simulink model "tgov1"  (R2014b)
settings: Solver=ode4  StartTime=0.0  StopTime=30  FixedStep=30/100  RelTol=1e-3  EnableMultiTasking=on
values from neighbouring files (symbols this model uses):
  delta_w = 0.0    (= 0)    [tgov1_test.m]
  Dt = 0.0    (= 0)    [tgov1_test.m]
  Pref = .50    (= 0.5)    [tgov1_test.m]
  R = 0.05    [tgov1_test.m]
  T1 = 0.5    [tgov1_test.m]
  T2 = 3.0    (= 3)    [tgov1_test.m]
  T3 = 10.0    (= 10)    [tgov1_test.m]
settings Model: Creator=thad  LastModifiedBy=heyth
settings OptimizationCC: UseDivisionForNetSlopeComputation=off  SimCompilerOptimization=off
settings DebuggingCC: FcnCallInpInsideContextMsg=error  FrameProcessingCompatibilityMsg=error  SFExecutionAtInitializationDiag=none
settings HardwareCC: ProdBitPerSizeT=32  ProdBitPerPtrDiffT=32
settings RTWCC: RTWCompilerOptimization=off
settings ConfigComp: CovMetricSettings=dw  CovHtmlReporting=on  CovSaveCumulativeToWorkspaceVar=on  CovSaveSingleToWorkspaceVar=on  CovExternalEMLEnable=off  CovSFcnEnable=off

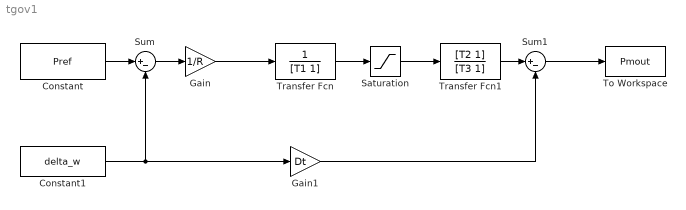
== system tgov1 ==
  Constant : Constant  Value=Pref
  Constant1 : Constant  Value=delta_w
  Gain : Gain  Gain=1/R
  Gain1 : Gain  Gain=Dt
  Saturation : Saturate  UpperLimit=1  LowerLimit=0
  Sum : Sum  Inputs=|+-
  Sum1 : Sum  Inputs=|+-
  To Workspace : ToWorkspace  VariableName=Pmout  SampleTime=-1
  Transfer Fcn : TransferFcn  Denominator=[T1 1]
  Transfer Fcn1 : TransferFcn  Numerator=[T2 1]  Denominator=[T3 1]
  wires:
  Constant1/1 -> Sum/2, Gain1/1
  Transfer Fcn/1 -> Saturation/1
  Saturation/1 -> Transfer Fcn1/1
  Gain1/1 -> Sum1/2
  Transfer Fcn1/1 -> Sum1/1
  Sum1/1 -> To Workspace/1
  Constant/1 -> Sum/1
  Sum/1 -> Gain/1
  Gain/1 -> Transfer Fcn/1
